simulink model "first"  (R2022b)
settings: Solver=VariableStepAuto  StartTime=0.0  StopTime=100  RelTol=1e-3
settings Model: Creator=zuzanna  LastModifiedBy=zuzanna

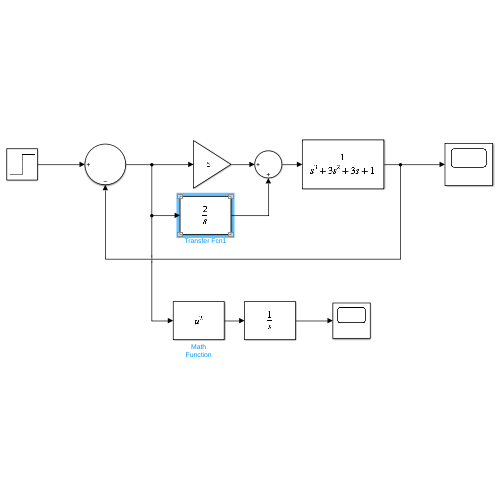
[thumbnail: Simulink's stored preview of the top-level diagram]
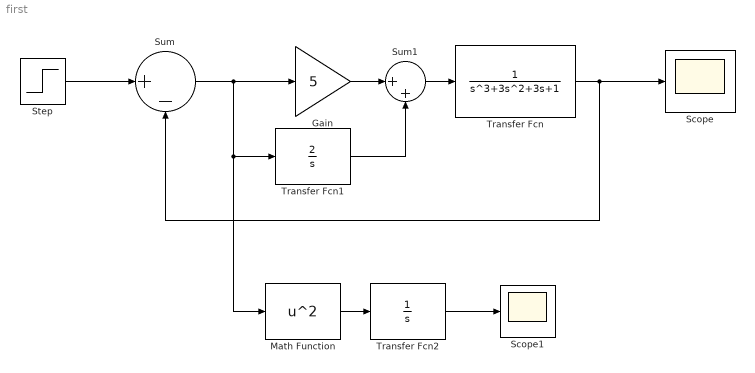
== system first ==
  Gain : Gain  Gain=5
  Math Function : Math  Operator=square
  Scope : Scope
  Scope1 : Scope
  Step : Step  SampleTime=0
  Sum : Sum  Inputs=|+-
  Sum1 : Sum  Inputs=|++
  Transfer Fcn : TransferFcn  Denominator=[1 3 3 1]
  Transfer Fcn1 : TransferFcn  Numerator=[2]  Denominator=[1 0]
  Transfer Fcn2 : TransferFcn  Denominator=[1 0]
  wires:
  Sum/1 -> Math Function/1, Transfer Fcn1/1, Gain/1
  Transfer Fcn/1 -> Scope/1, Sum/2
  Step/1 -> Sum/1
  Transfer Fcn1/1 -> Sum1/2
  Gain/1 -> Sum1/1
  Sum1/1 -> Transfer Fcn/1
  Math Function/1 -> Transfer Fcn2/1
  Transfer Fcn2/1 -> Scope1/1
